simulink model "p_ctrl"  (R2020a)
settings: Solver=ode45  StartTime=0.0  StopTime=50  MaxStep=1e-3  RelTol=1e-3
libraries: simulink x1
settings Model: Creator=Csurleny  LastModifiedBy=Csurleny

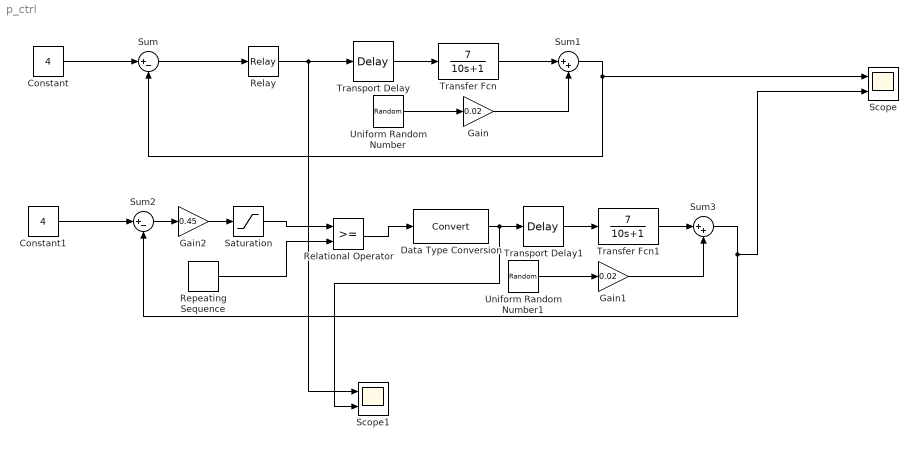
== system p_ctrl ==
  Constant : Constant  Value=4
  Constant1 : Constant  Value=4
  Data Type Conversion : DataTypeConversion
  Gain : Gain  Gain=0.02
  Gain1 : Gain  Gain=0.02
  Gain2 : Gain  Gain=0.45
  Relational Operator : RelationalOperator  OutDataTypeStr=boolean  RndMeth=Simplest
  Relay : Relay  OnSwitchValue=0.02  OffSwitchValue=-0.02
  Repeating Sequence : simulink/Sources/Repeating Sequence  rep_seq_t=[0 0.5]  rep_seq_y=[0 1]
  Saturation : Saturate  UpperLimit=1  LowerLimit=0
  Scope : Scope  NumInputPorts=2
  Scope1 : Scope  NumInputPorts=2
  Sum : Sum  Inputs=|+-
  Sum1 : Sum  Inputs=|++
  Sum2 : Sum  Inputs=|+-
  Sum3 : Sum  Inputs=|++
  Transfer Fcn : TransferFcn  Numerator=[7]  Denominator=[10 1]
  Transfer Fcn1 : TransferFcn  Numerator=[7]  Denominator=[10 1]
  Transport Delay : TransportDelay  DelayTime=3
  Transport Delay1 : TransportDelay  DelayTime=3
  Uniform Random Number : UniformRandomNumber  SampleTime=0.1
  Uniform Random Number1 : UniformRandomNumber  SampleTime=0.1
  wires:
  Transfer Fcn/1 -> Sum1/1
  Uniform Random Number/1 -> Gain/1
  Relay/1 -> Scope1/1, Transport Delay/1
  Sum1/1 -> Scope/1, Sum/2
  Constant/1 -> Sum/1
  Sum/1 -> Relay/1
  Transport Delay/1 -> Transfer Fcn/1
  Gain/1 -> Sum1/2
  Constant1/1 -> Sum2/1
  Transport Delay1/1 -> Transfer Fcn1/1
  Gain1/1 -> Sum3/2
  Uniform Random Number1/1 -> Gain1/1
  Sum2/1 -> Gain2/1
  Sum3/1 -> Sum2/2, Scope/2
  Transfer Fcn1/1 -> Sum3/1
  Gain2/1 -> Saturation/1
  Saturation/1 -> Relational Operator/1
  Repeating Sequence/1 -> Relational Operator/2
  Data Type Conversion/1 -> Scope1/2, Transport Delay1/1
  Relational Operator/1 -> Data Type Conversion/1
